simulink library "INT_WESDem_StrtBtnSP"  (R2016b)
settings: Solver=VariableStepAuto  StartTime=0.0  StopTime=10.0  RelTol=1e-3
settings Model: Creator=zhoukai  LastModifiedBy=zhoukai

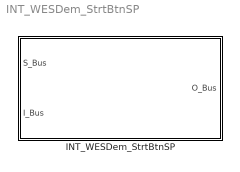
== system INT_WESDem_StrtBtnSP ==
  INT_WESDem_StrtBtnSP : Subsystem

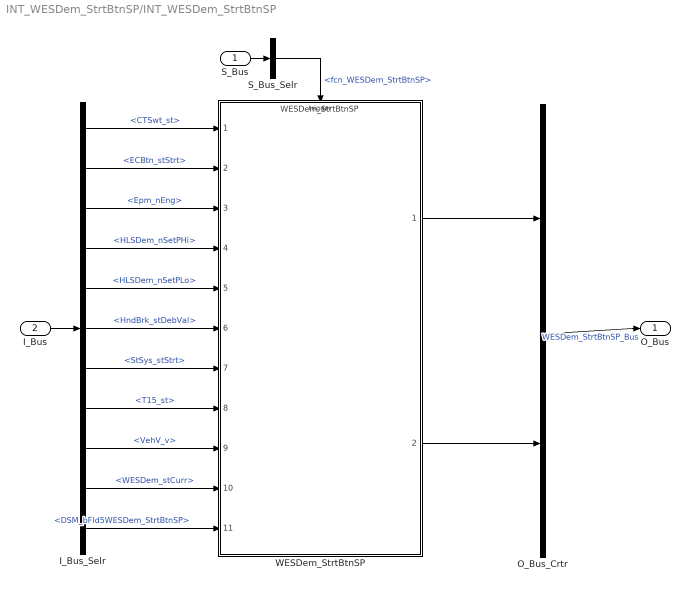
== system INT_WESDem_StrtBtnSP/INT_WESDem_StrtBtnSP ==
  S_Bus : Inport
  I_Bus : Inport  Port=2
  I_Bus_Selr : BusSelector  OutputSignals=CTSwt_st,ECBtn_stStrt,Epm_nEng,HLSDem_nSetPHi,HLSDem_nSetPLo,HndBrk_stDebVal,StSys_stStrt,T15_st,VehV_v,WESDem_stCurr,DSM_bFld5WESDem_StrtBtnSP
  O_Bus_Crtr : BusCreator  Inputs=2
  S_Bus_Selr : BusSelector  OutputSignals=fcn_WESDem_StrtBtnSP
  WESDem_StrtBtnSP : ModelReference  ModelNameDialog=WESDem_StrtBtnSP  SimulationMode=Normal  ModelReferenceVersion=1.23  TriggerPortName=function  TriggerPortTriggerType=function-call  TriggerPortStatesWhenEnabling=held
  O_Bus : Outport
  wires:
  S_Bus_Selr/1 -> WESDem_StrtBtnSP/Trigger  "<fcn_WESDem_StrtBtnSP>"
  S_Bus/1 -> S_Bus_Selr/1
  I_Bus/1 -> I_Bus_Selr/1
  I_Bus_Selr/1 -> WESDem_StrtBtnSP/1  "<CTSwt_st>"
  I_Bus_Selr/2 -> WESDem_StrtBtnSP/2  "<ECBtn_stStrt>"
  I_Bus_Selr/3 -> WESDem_StrtBtnSP/3  "<Epm_nEng>"
  I_Bus_Selr/4 -> WESDem_StrtBtnSP/4  "<HLSDem_nSetPHi>"
  I_Bus_Selr/5 -> WESDem_StrtBtnSP/5  "<HLSDem_nSetPLo>"
  I_Bus_Selr/6 -> WESDem_StrtBtnSP/6  "<HndBrk_stDebVal>"
  I_Bus_Selr/7 -> WESDem_StrtBtnSP/7  "<StSys_stStrt>"
  I_Bus_Selr/8 -> WESDem_StrtBtnSP/8  "<T15_st>"
  I_Bus_Selr/9 -> WESDem_StrtBtnSP/9  "<VehV_v>"
  I_Bus_Selr/10 -> WESDem_StrtBtnSP/10  "<WESDem_stCurr>"
  I_Bus_Selr/11 -> WESDem_StrtBtnSP/11  "<DSM_bFld5WESDem_StrtBtnSP>"
  O_Bus_Crtr/1 -> O_Bus/1  "WESDem_StrtBtnSP_Bus"
  WESDem_StrtBtnSP/1 -> O_Bus_Crtr/1
  WESDem_StrtBtnSP/2 -> O_Bus_Crtr/2
